simulink model "USV_NEW"  (R2025b)
settings: Solver=ode45  StartTime=0.0  StopTime=1000  RelTol=1e-4  AbsTol=1e-6
settings Model: Creator=Juanjose  LastModifiedBy=Juanjose

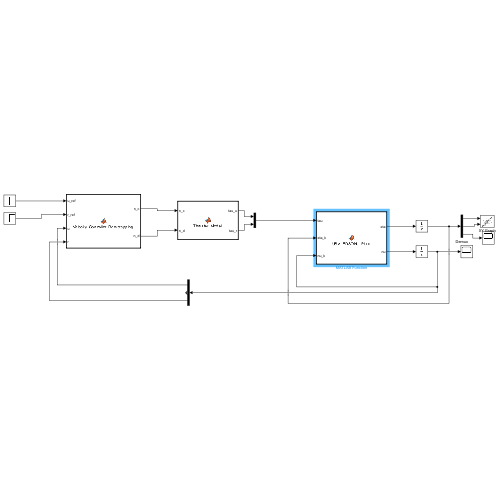
[thumbnail: Simulink's stored preview of the top-level diagram]
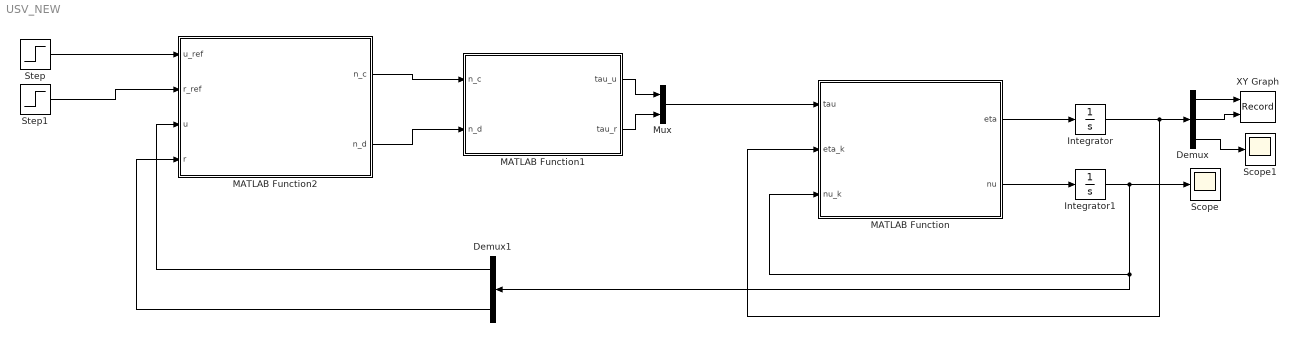
== system USV_NEW ==
  Demux : Demux  Outputs=3
  Demux1 : Demux  Outputs=3
  Integrator : Integrator  InitialCondition=[0.001; 0.001; 0.001]
  Integrator1 : Integrator  InitialCondition=[0.001; 0.001; 0.001]
  MATLAB Function : MATLAB Function  TreatAsAtomicUnit=on
  MATLAB Function1 : MATLAB Function  TreatAsAtomicUnit=on
  MATLAB Function2 : MATLAB Function  TreatAsAtomicUnit=on
  Mux : Mux  Inputs=2
  Scope : Scope
      settings: ActiveDisplayYMinimum=-0.30627013477746645  ActiveDisplayYMaximum=1.3626376945694334
  Scope1 : Scope
      settings: ActiveDisplayYMinimum=-7.4719126455864258  ActiveDisplayYMaximum=67.257213810277847
  Step : Step  After=2  SampleTime=0
  Step1 : Step  After=0.5  SampleTime=0
  XY Graph : Record  NumPorts=2.0  FileSettingsInternal="{\"entries\":[{\"content\":{\"excelSettings\":{\"content\":{},\"type\":\"Streamout.ExcelSettings\"},\"parquetSettings\":{\"content\":{},\"type\":\"Streamout.ParquetSettings\"}},\"type\":\"Streamout.FileSettingStorage\",\"uuid\":\"\"}],\"packageUris\":[\"http:\\/\\/schema.mathworks.com\\/mf0\\/streamout_blocks\\/R2020a\"],\"version\":\"1.0\"}"  FrameSettings=[0, 0]  Layout=[1 1]  SignalsInternal="{\"entries\":[{\"content\":{\"signals\":[{\"content\":{\"blockPath\":[],\"dimensions\":[1],\"domain\":\"\",\"lineColor\":\"#a2142f\",\"plots\":[ 1 ],\"port\":1,\"sid\":[\"\"],\"signalID\":1,\"signalName\":\"Demux:1\"},\"type\":\"RecordBlkView.Signal\",\"uuid\":\"\"},{\"content\":{\"blockPath\":[],\"dimensions\":[1],\"domain\":\"\",\"lineColor\":\"#139fff\",\"plots\":[ 1 ],\"port\":2,\"sid\":[\"\"],\"signalID\":2,\"signalName\":\"Demux:2\"},\"type\":\"RecordBlkView.Signal\",\"uuid\":\"\"}]},\"type\":\"RecordBlkView.InputSignals\",\"uuid\":\"\"}],\"packageUris\":[\"http:\\/\\/schema.mathworks.com\\/mf0\\/streamout_blocks\\/R2020a\"],\"version\":\"1.0\"}"  VisualizationBindings="{\"xyplotplugin\":{\"info\":[{\"series\":[{\"bindingParametersList\":[{\"parameter\":\"X-Axis\",\"signalID\":1,\"signalName\":\"Demux:1\"},{\"parameter\":\"Y-Axis\",\"signalID\":2,\"signalName\":\"Demux:2\"}],\"seriesID\":0}],\"subplotID\":1}]}}"  CompatibilityTag=XY
  wires:
  MATLAB Function/1(eta) -> Integrator/1
  MATLAB Function/2(nu) -> Integrator1/1
  Integrator1/1 -> Scope/1, Demux1/1, MATLAB Function/3(nu_k)
  Integrator/1 -> MATLAB Function/2(eta_k), Demux/1
  Demux/1 -> XY Graph/1
  Demux/2 -> XY Graph/2
  Demux/3 -> Scope1/1
  MATLAB Function1/2(tau_r) -> Mux/2
  MATLAB Function1/1(tau_u) -> Mux/1
  Mux/1 -> MATLAB Function/1(tau)
  MATLAB Function2/1(n_c) -> MATLAB Function1/1(n_c)
  MATLAB Function2/2(n_d) -> MATLAB Function1/2(n_d)
  Demux1/1 -> MATLAB Function2/3(u)
  Step/1 -> MATLAB Function2/1(u_ref)
  Demux1/3 -> MATLAB Function2/4(r)
  Step1/1 -> MATLAB Function2/2(r_ref)

== matlab function USV_NEW/MATLAB Function1 ==
  data: n_c input; tau_u output; n_d input; tau_r output
function [tau_u, tau_r] = Thruster_Model(n_c, n_d)
%#codegen
% Propulsión diferencial (dos MinnKota). n_c=(n1+n2)/2, n_d=(n1-n2)/2

%% Geometría y fluido
Dp = 0.15;           % [m] diámetro hélice
rho = 1025;          % [kg/m^3] agua de mar
B   = 1.6;           % [m] manga del catamarán
lever = B/2;         % [m] brazo de palanca yaw

%% Coeficientes polinomiales KT(J) y KQ(J) (si solo usas KT basta)
a0 = 0.1884;  a1 = -0.1507;  a2 = -0.1132;  % KT
% b0 = 0.0113; b1 = -0.0325;  b2 = -0.0102; % KQ (no usado aquí)
u_current = 0;
%% Saturación de velocidades
n_max = 22;                      % [rps]
n_c = max(min(n_c, n_max), -n_max);
n_d = max(min(n_d, n_max/2), -n_max/2);

%% Reconstrucción de rotores
n1 = n_c + n_d;
n2 = n_c - n_d;

%% Advance ratio J = u_rel / (n*D)
% u_current es la velocidad relativa del flujo en el disco (ver sección 5)
if abs(n1) > 1e-6, J1 = u_current/(n1*Dp); else, J1 = 0; end
if abs(n2) > 1e-6, J2 = u_current/(n2*Dp); else, J2 = 0; end

KT1 = a2*J1*J1 + a1*J1 + a0;
KT2 = a2*J2*J2 + a1*J2 + a0;

% Empuje T = KT * rho * n^2 * D^4
T1 = KT1 * rho * (n1*n1) * (Dp^4);
T2 = KT2 * rho * (n2*n2) * (Dp^4);

%% Resultantes en el cuerpo
tau_u = T1 + T2;
tau_r = (T1 - T2) * lever;
end

== matlab function USV_NEW/MATLAB Function ==
  data: tau input; eta output; eta_k input; nu_k input; nu output
function [eta, nu] = USV_EDSONJ_Plant(tau, eta_k, nu_k)
% =========================================================================
% Planta USV EDSON-J 3-DOF - CORREGIDO según matrices del artículo
% =========================================================================
% ENTRADAS:
%   tau   : [2x1] = [tau_u; tau_r] → Fuerza surge y momento yaw
%   eta_k : [3x1] = [x; y; psi]    → Estado de posición
%   nu_k  : [3x1] = [u; v; r]      → Estado de velocidad
%
% SALIDAS:
%   eta : [3x1] = derivada de posición
%   nu  : [3x1] = derivada de velocidad
% =========================================================================

%% ========== PARÁMETROS FÍSICOS ==========================================
m  = 250.0;         % [kg]
Iz = 201.1;         % [kg·m²]
xg = 0.11;          % [m]

%% ========== COEFICIENTES HIDRODINÁMICOS (Tabla 2) =======================
% Masa añadida
Xu_dot = -2.471;    % [kg]
Yv_dot = -247.065;  % [kg]
Yr_dot = -370.597;  % [kg·m]
Nv_dot = -370.597;  % [kg·m]
Nr_dot = -748.310;  % [kg·m²]

% Amortiguamiento lineal
Xu = -0.291;        % [kg/s]
Yv = -123.532;      % [kg/s]
Nr = -741.195;      % [kg·m²/s]

% Amortiguamiento cuadrático
Xuu = -27.626;      % [kg/m]
Yvv = -38.928;      % [kg/m]
Nrr = -262.791;     % [kg·m²/rad²]

%% ========== MATRIZ DE INERCIA M =========================================
M11 = m - Xu_dot;
M22 = m - Yv_dot;
M23 = m*xg - Yr_dot;
M32 = m*xg - Nv_dot;
M33 = Iz - Nr_dot;

M = [M11,  0,    0;
     0,    M22,  M23;
     0,    M32,  M33];

%% ========== MATRIZ DE CORIOLIS C(nu) ====================================
u = nu_k(1); 
v = nu_k(2); 
r = nu_k(3);

CRB = [  0,   -m*r,     -m*xg*r;
        m*r,    0,           0;
      m*xg*r,   0,           0];

CA  = [  0,     0,       Yv_dot*v + Yr_dot*r;
         0,     0,      -Xu_dot*u;
       -Yv_dot*v - Yr_dot*r,  Xu_dot*u,  0];

C = CRB + CA;

%% ========== MATRIZ DE AMORTIGUAMIENTO D(nu) =============================
D11 = Xu + Xuu*abs(u);
D22 = Yv + Yvv*abs(v);
D33 = Nr + Nrr*abs(r);

D = -diag([D11, D22, D33]);

%% ========== DINÁMICA ====================================================
tau_full = [tau(1); 0; tau(2)];
nu_dot = M \ (tau_full - C*nu_k - D*nu_k);

%% ========== CINEMÁTICA ==================================================
psi = eta_k(3);
J = [cos(psi), -sin(psi), 0;
     sin(psi),  cos(psi), 0;
     0,         0,        1];

eta_dot = J * nu_k;

%% ========== SALIDAS ======================================================
eta = eta_dot;
nu  = nu_dot;

end

== matlab function USV_NEW/MATLAB Function2 ==
  data: u_ref input; n_c output; r_ref input; u input; n_d output; r input
function [n_c, n_d] = Velocity_Controller_Backstepping(u_ref, r_ref, u, r)
%#codegen
% Backstepping básico en velocidades (surge/yaw).
% Salida: n_c, n_d (rps) para alimentar Thruster_Model

%% --- Parámetros (de la planta/propulsor) ---
% Hidrodinámica (coincidir con planta)
Xu = -0.291;   Xuu = -27.626;
Nr = -741.195; Nrr = -262.791;

% Hélice/fluido
Dp = 0.15;  rho = 1025;  a0 = 0.1884;   % KT ~ a0 cerca de J≈0
B  = 1.6;   lever = B/2; nmax = 22;

%% --- Errores ---
zu = u - u_ref;
zr = r - r_ref;

%% --- Fricción principal (compensación “d_u/d_r”) ---
d_u = (Xu  + Xuu*abs(u))*u;   % signo ya coherente con planta
d_r = (Nr  + Nrr*abs(r))*r;

%% --- Ley de control (forma simple regulatoria) ---
k_u1 = 80;  k_u2 = 40;
k_r1 = 80;  k_r2 = 50;

tau_u = -k_u1*zu - k_u2*tanh(zu) - d_u;   % suave y robusta
tau_r = -k_r1*zr - k_r2*tanh(zr) - d_r;

%% --- Asignación a rotores: T1/2 desde tau_u, tau_r ---
T1 = 0.5*tau_u + tau_r/lever;
T2 = 0.5*tau_u - tau_r/lever;

% Inversa abierta (KT≈a0): n = sign(T)*sqrt(|T|/(KT*rho*D^4))
KT1 = a0; KT2 = a0;
n1 = 0; n2 = 0;
if T1 ~= 0
    n1 = sign(T1)*sqrt( max(0,abs(T1)) / (KT1*rho*(Dp^4)) );
end
if T2 ~= 0
    n2 = sign(T2)*sqrt( max(0,abs(T2)) / (KT2*rho*(Dp^4)) );
end

% Modo común / diferencial + saturación
n_c = (n1 + n2)/2;
n_d = (n1 - n2)/2;
n_c = max(min(n_c, nmax), -nmax);
n_d = max(min(n_d, nmax/2), -nmax/2);
end
